simulink model "signal_dvPrivate_acMethod"  (R2024b)
settings: configuration reference "model_cfg" (kept outside this file)
model workspace (MATLAB code in the model file):
  | cmdLim = Simulink.Parameter;
  | cmdLim.Value = 15;
  | cmdLim.Description = 'Limit for controlling the maximum surface command angle.';
  | cmdLim.Min = 0;
  | cmdLim.Max = 90;
  | cmdLim.DocUnits = 'deg';
  | 
  | dispGain = Simulink.Parameter;
  | dispGain.Value = 0.75;
  | dispGain.Description = 'Gain applied to the displacement error.';
  | dispGain.Min = 0;
  | dispGain.Max = [];
  | dispGain.DocUnits = 'deg/sec/deg';
  | 
  | dispLim = Simulink.Parameter;
  | dispLim.Value = 30;
  | dispLim.Description = 'Limit for controlling the maximum commanded angle.';
  | dispLim.Min = 0;
  | dispLim.Max = 180;
  | dispLim.DocUnits = 'deg';
  | 
  | intGain = Simulink.Parameter;
  | intGain.Value = 0.5;
  | intGain.Description = 'Gain applied to the integral error.';
  | intGain.Min = 0;
  | intGain.Max = [];
  | intGain.DocUnits = 'deg/sec/deg/sec';
  | 
  | intLim = Simulink.Parameter;
  | intLim.Value = 5;
  | intLim.Description = 'Limit for controlling the maximum commanded angle.';
  | intLim.Min = 0;
  | intLim.Max = 90;
  | intLim.DocUnits = 'deg';
  | 
  | rateGain = Simulink.Parameter;
  | rateGain.Value = 2;
  | rateGain.Description = 'Gain applied to the rate error.';
  | rateGain.Min = 0;
  | rateGain.Max = [];
  | rateGain.DocUnits = 'deg/deg/sec';
  | 
  | rateLim = Simulink.Parameter;
  | rateLim.Value = 6;
  | rateLim.Description = 'Limit for controlling the maximum commanded angle.';
  | rateLim.Min = 0;
  | rateLim.Max = 180;
  | rateLim.DocUnits = 'deg/sec';
  | 
  | hdgGain = Simulink.Parameter;
  | hdgGain.Value = 0.015;
undefined symbols (not defined in the file or in its folder): ParamArray, ParamScalar
settings Model: RequirementInfo={} %GIDa_fe9045fd_0412_4b6e_8206_617cc20e6fde  Creator=nabilekhoury  LastModifiedBy=nabilekhoury
settings ConfigSetRef: SourceName=model_cfg  SourceLocation=Base Workspace

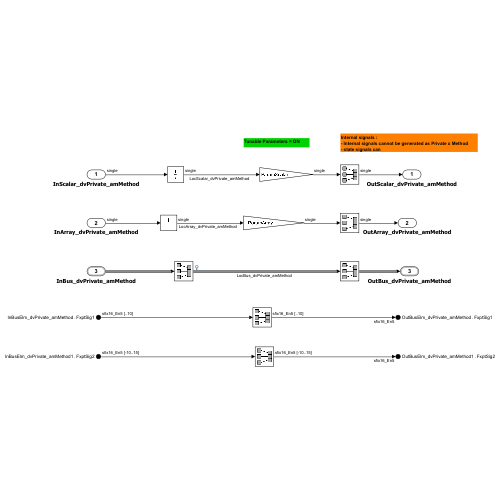
[thumbnail: Simulink's stored preview of the top-level diagram]
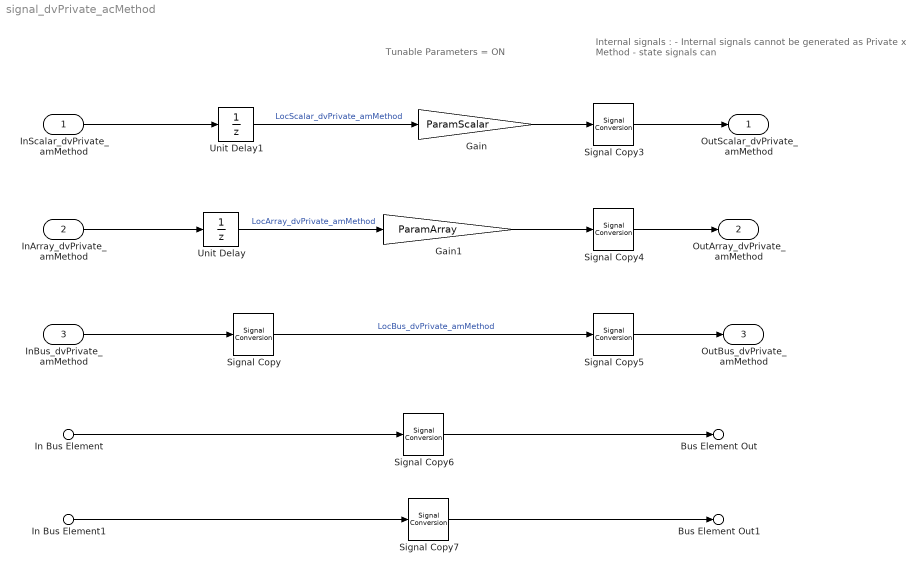
== system signal_dvPrivate_acMethod ==
  note: Tunable Parameters = ON
  note: Internal signals :
      | - Internal signals cannot be generated as Private x Method
      | - state signals can
  InScalar_dvPrivate_amMethod : Inport  OutDataTypeStr=single
  InArray_dvPrivate_amMethod : Inport  Port=2  OutDataTypeStr=single  PortDimensions=2
  InBus_dvPrivate_amMethod : Inport  Port=3  OutDataTypeStr=Bus: myBus
  In Bus Element : Inport  Port=4  PortName=InBusElm_dvPrivate_amMethod  Element=FxptSig1
  In Bus Element1 : Inport  Port=5  PortName=InBusElm_dvPrivate_amMethod1  Element=FxptSig2
  Gain : Gain  Gain=ParamScalar
  Gain1 : Gain  Gain=ParamArray
  Signal Copy{,3..7} (6 alike) : SignalConversion  OverrideOpt=off
  Unit Delay : UnitDelay  SampleTime=-1  StateName=LocArray_dvPrivate_amMethod  HasFrameUpgradeWarning=on
  Unit Delay1 : UnitDelay  SampleTime=-1  StateName=LocScalar_dvPrivate_amMethod  HasFrameUpgradeWarning=on
  OutScalar_dvPrivate_amMethod : Outport  VectorParamsAs1DForOutWhenUnconnected=off
  OutArray_dvPrivate_amMethod : Outport  Port=2  PortDimensions=2  VectorParamsAs1DForOutWhenUnconnected=off
  OutBus_dvPrivate_amMethod : Outport  Port=3  OutDataTypeStr=Bus: myBus  VectorParamsAs1DForOutWhenUnconnected=off
  Bus Element Out : Outport  Port=4  PortName=OutBusElm_dvPrivate_amMethod  Element=FxptSig1
  Bus Element Out1 : Outport  Port=5  PortName=OutBusElm_dvPrivate_amMethod1  Element=FxptSig2
  wires:
  InScalar_dvPrivate_amMethod/1 -> Unit Delay1/1
  Unit Delay1/1 -> Gain/1  "LocScalar_dvPrivate_amMethod"
  InArray_dvPrivate_amMethod/1 -> Unit Delay/1
  Unit Delay/1 -> Gain1/1  "LocArray_dvPrivate_amMethod"
  InBus_dvPrivate_amMethod/1 -> Signal Copy/1
  Signal Copy/1 -> Signal Copy5/1  "LocBus_dvPrivate_amMethod"
  Signal Copy3/1 -> OutScalar_dvPrivate_amMethod/1
  Signal Copy4/1 -> OutArray_dvPrivate_amMethod/1
  Signal Copy5/1 -> OutBus_dvPrivate_amMethod/1
  In Bus Element/1 -> Signal Copy6/1
  Signal Copy6/1 -> Bus Element Out/1
  Gain/1 -> Signal Copy3/1
  Gain1/1 -> Signal Copy4/1
  Signal Copy7/1 -> Bus Element Out1/1
  In Bus Element1/1 -> Signal Copy7/1
